simulink model "coverage_control"  (R2025b)
settings: Solver=FixedStepAuto  StartTime=0.0  StopTime=t_end  FixedStep=dt  RelTol=1e-3
undefined symbols (not defined in the file): coverage_region, k, p_init
settings Model: Creator=yamauchi  LastModifiedBy=01

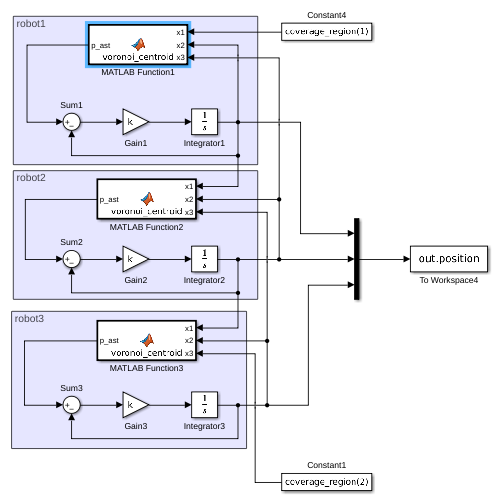
[thumbnail: Simulink's stored preview of the top-level diagram]
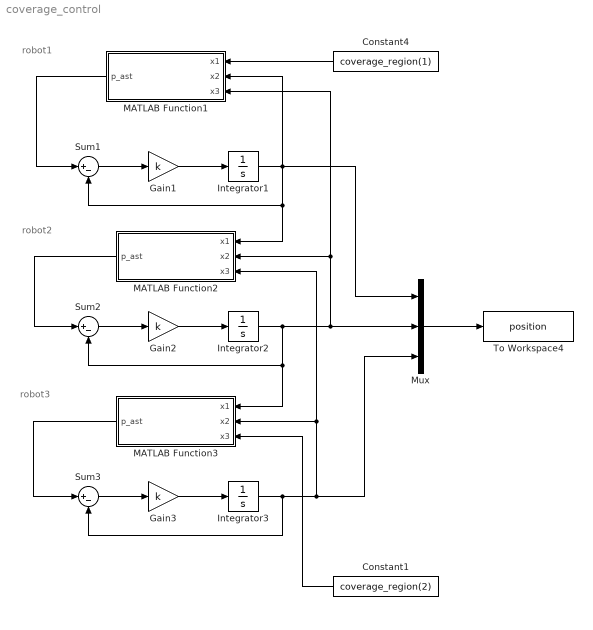
== system coverage_control ==
  note: robot3
  note: robot2
  note: robot1
  Constant1 : Constant  Value=coverage_region(2)
  Constant4 : Constant  Value=coverage_region(1)
  Gain1 : Gain  Gain=k
  Gain2 : Gain  Gain=k
  Gain3 : Gain  Gain=k
  Integrator1 : Integrator  InitialCondition=p_init(1)
  Integrator2 : Integrator  InitialCondition=p_init(2)
  Integrator3 : Integrator  InitialCondition=p_init(3)
  MATLAB Function1 : MATLAB Function  TreatAsAtomicUnit=on
  MATLAB Function2 : MATLAB Function  TreatAsAtomicUnit=on
  MATLAB Function3 : MATLAB Function  TreatAsAtomicUnit=on
  Mux : Mux  Inputs=3
  Sum1 : Sum  Inputs=|+-
  Sum2 : Sum  Inputs=|+-
  Sum3 : Sum  Inputs=|+-
  To Workspace4 : ToWorkspace  VariableName=position  SampleTime=-1
      settings: Save2DSignal=2-D array (concatenate along first dimension)
  wires:
  Sum1/1 -> Gain1/1
  Integrator1/1 -> MATLAB Function1/2(x2), Mux/1, MATLAB Function2/1(x1), Sum1/2
  MATLAB Function1/1(p_ast) -> Sum1/1
  Gain1/1 -> Integrator1/1
  Sum2/1 -> Gain2/1
  Integrator2/1 -> Mux/2, MATLAB Function1/3(x3), MATLAB Function2/2(x2), MATLAB Function3/1(x1), Sum2/2
  MATLAB Function2/1(p_ast) -> Sum2/1
  Gain2/1 -> Integrator2/1
  Gain3/1 -> Integrator3/1
  MATLAB Function3/1(p_ast) -> Sum3/1
  Integrator3/1 -> MATLAB Function2/3(x3), MATLAB Function3/2(x2), Mux/3, Sum3/2
  Sum3/1 -> Gain3/1
  Constant4/1 -> MATLAB Function1/1(x1)
  Constant1/1 -> MATLAB Function3/3(x3)
  Mux/1 -> To Workspace4/1

== matlab function coverage_control/MATLAB Function3 ==
  data: x1 input; p_ast output; x2 input; x3 input
function p_ast = voronoi_centroid(x1, x2, x3)

a = (x1 + x2)/2;
b = x3;

p_ast = (3/4)*((b^4 - a^4)/(b^3 - a^3));

== matlab function coverage_control/MATLAB Function1 ==
  data: x1 input; p_ast output; x2 input; x3 input
function p_ast = voronoi_centroid(x1, x2, x3)
a = x1;
b = (x2 + x3)/2;

p_ast = (3/4)*((b^4 - a^4)/(b^3 - a^3));

== matlab function coverage_control/MATLAB Function2 ==
  data: x1 input; p_ast output; x2 input; x3 input
function p_ast = voronoi_centroid(x1, x2, x3)

a = (x1 + x2)/2;
b = (x2 + x3)/2;

p_ast = (3/4)*((b^4 - a^4)/(b^3 - a^3));
